simulink model "Grid_PBFORCAPF_ab_Detail_2013b_616"  (R2021b)
settings: Solver=FixedStepDiscrete  StartTime=0.0  StopTime=1.5  FixedStep=Ts_Power  RelTol=1e-3
InitFcn:
  | %% Sys Para
  | N=200;fg=50;Vbase=200;
  | Ts_Control=1/N/fg;
  | Tscon=Ts_Control;
  | Ts_Power=Ts_Control/128;
  | fsw=1/Ts_Control;
  | Vdcref=350;
  | Vdcini=Vdcref;
  | 
  | 
  | 
  | %% Load Side
  | Ll=2.0e-3;Rl=1e-2;
  | RL=100;
  | 
  | %% DG Circuit Parameters
  | %% LCL
  | L1_DG1=1.4e-3;R1=1e-3;
  | L2_DG1=0.4e-3;R2=1e-3;
  | Cx_DG1=6.3e-6;
  | 
  | L1_DG2=L1_DG1;L2_DG2=L2_DG1;Cx_DG2=Cx_DG1;
  | L1_DG3=L1_DG1;L2_DG3=L2_DG1;Cx_DG3=Cx_DG1;
  | Cdc=0.55e-3;
  | %PLL;
  | Kp_pll=88;
  | Ki_pll=0.4/Ts_Control;
  | 
  | %% DG2 Controller Parameters
  | Kpc_DG1=4.89;
  | Kic_DG1=0;
  | 
  | Kpdc_DG1=0.2;
  | Kidc_DG1=0.1;
undefined symbols (not defined in the file or in its folder): DiscIntNeverNeededParam, L2, Rd
libraries: spsThreePhaseSeriesRLCBranchLib x13, slpidlib x8, spsThreePhaseVIMeasurementLib x8, spsStairGeneratorLib x8, simulink x6, simulink_extras x6, spsSeriesRLCBranchLib x5, spsThreePhaseBreakerLib x5, spsUniversalBridgeLib x4, spsNeutralLib x4, spsGroundLib x3, spsPWMGenerator2LevelLib x3
(part 2 of 3)

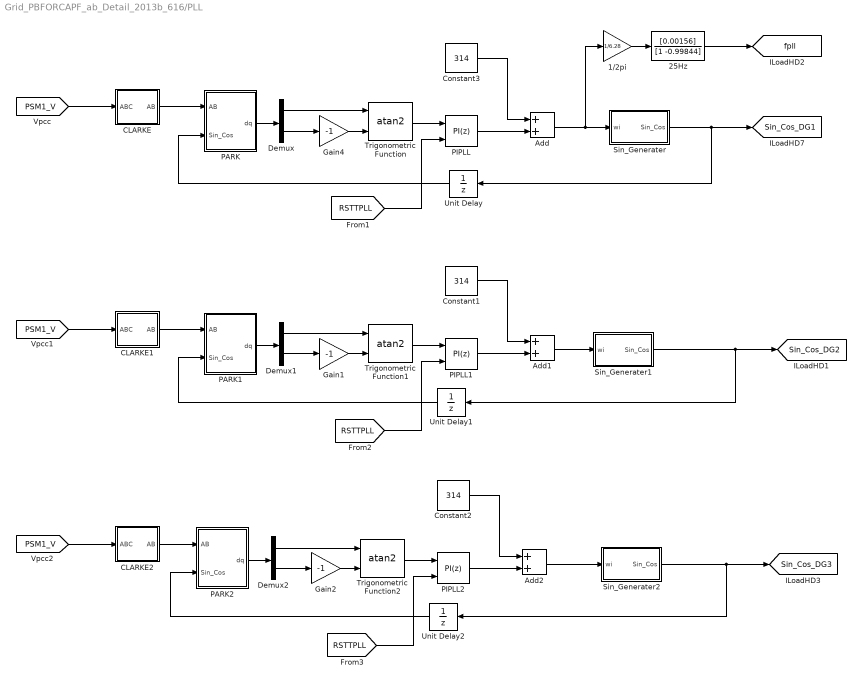
== system Grid_PBFORCAPF_ab_Detail_2013b_616/PLL ==
  1/2pi : Gain  Gain=1/6.28
  25Hz : DiscreteFilter  Numerator=[0.00156]  Denominator=[1 -0.99844]  InitialStates=50  InputProcessing=Columns as channels (frame based)  FilterStructure=Direct form II transposed
  Add : Sum
  Add1 : Sum
  Add2 : Sum
  CLARKE : Subsystem
  CLARKE1 : Subsystem
  CLARKE2 : Subsystem
  Constant1 : Constant  Value=314  SampleTime=Tscon
  Constant2 : Constant  Value=314  SampleTime=Tscon
  Constant3 : Constant  Value=314  SampleTime=Tscon
  Demux : Demux  Outputs=2
  Demux1 : Demux  Outputs=2
  Demux2 : Demux  Outputs=2
  Gain1 : Gain  Gain=-1
  Gain2 : Gain  Gain=-1
  Gain4 : Gain  Gain=-1
  PARK : Subsystem
  PARK1 : Subsystem
  PARK2 : Subsystem
  PIPLL : slpidlib/PID Controller  Controller=PI  Form=Parallel  TimeDomain=Discrete-time  UseExternalTs=off  SampleTime=-1  IntegratorMethod=Backward Euler  FilterMethod=Forward Euler  ControllerParametersSource=internal  P=Kp_pll  I=Ki_pll  D=0  N=100  UseFilter=on  TunerSelectOption=Transfer Function Based (PID Tuner App)  InitialConditionSource=internal  InitialConditionForIntegrator=0  InitialConditionForFilter=0  DifferentiatorICPrevScaledInput=0  ExternalReset=level  TrackingMode=off  Kt=1  LimitOutput=on  SatLimitsSource=internal  UpperSaturationLimit=100  LowerSaturationLimit=-100  LinearizeAsGain=off  AntiWindupMode=none  Kb=0.5  POutMin=[]  POutMax=[]  IOutMin=[]  IOutMax=[]  DOutMin=[]  DOutMax=[]  NOutMin=[]  NOutMax=[]  SumOutMin=[]  SumOutMax=[]  SaturationOutMin=[]  SaturationOutMax=[]  PParamMin=[]  PParamMax=[]  IParamMin=[]  IParamMax=[]  DParamMin=[]  DParamMax=[]  NParamMin=[]  NParamMax=[]  KbParamMin=[]  KbParamMax=[]  KtParamMin=[]  KtParamMax=[]  KbOutMin=[]  KbOutMax=[]  KtOutMin=[]  KtOutMax=[]  IntegratorOutMin=[]  IntegratorOutMax=[]  FilterOutMin=[]  FilterOutMax=[]  SumI1OutMin=[]  SumI1OutMax=[]  SumI2OutMin=[]  SumI2OutMax=[]  SumI3OutMin=[]  SumI3OutMax=[]  SumI4OutMin=[]  SumI4OutMax=[]  SumDOutMin=[]  SumDOutMax=[]  DifferentiatorOutMin=[]  DifferentiatorOutMax=[]  FilterDiffOutCoefMin=[]  FilterDiffOutCoefMax=[]  ReciprocalOutMin=[]  ReciprocalOutMax=[]  SumDenOutMin=[]  SumDenOutMax=[]  SumNumOutMin=[]  SumNumOutMax=[]  DivideOutMin=[]  DivideOutMax=[]  UdiffTsProdOutMin=[]  UdiffTsProdOutMax=[]  NTsProdOutMin=[]  NTsProdOutMax=[]  UintegralTsProdOutMin=[]  UintegralTsProdOutMax=[]  UngainTsProdOutMin=[]  UngainTsProdOutMax=[]  IntegratorContinuousStateAttributes=''  IntegratorStateMustResolveToSignalObject=off  IntegratorRTWStateStorageClass=Auto  FilterContinuousStateAttributes=''  FilterStateMustResolveToSignalObject=off  FilterRTWStateStorageClass=Auto  ParallelPVariant=InternalParameters  IdealPVariant=Disabled  IVariant=InternalParameters  DVariant=Disabled  IntegratorVariant=Discrete  SatVariant=Enabled  AWVariant=Passthrough  PCopyVariant=Disabled  TRVariant=Disabled  FdbkBlocksVariant=Forward  IdealPFdbkVariant=Disabled  SatFdbkVariant=Disabled  DerivativeFilterVariant=Disabled  NVariant=Disabled  NCopyVariant=Disabled_SignalSpec  FilterICVariant=Disabled  IntegratorICVariant=InternalICs  ExternalResetVariant=ExternalReset  TRSumVariant=Passthrough  SumFdbkVariant=Disabled  SumVariant=Sum_PI  TsampFilterVariant=InternalTs  TsampNgainVariant=Passthrough  TsampIntegralVariant=Passthrough  ExternalSaturationOutDataTypeStr=Inherit: Same as second input
      link override Integrator: IntegratorMethod=Integration: Backward Euler  gainval=1.0  ExternalReset=level  InitialConditionSource=internal  InitialCondition=InitialConditionForIntegrator  InitialConditionMode=State only (most efficient)  SampleTime=-1  OutMin=IntegratorOutMin  OutMax=IntegratorOutMax  OutDataTypeStr=IntegratorOutDataTypeStr  LimitOutput=off  UpperSaturationLimit=inf  LowerSaturationLimit=-inf  ShowSaturationPort=off  ShowStatePort=off
      link override Integrator: StateMustResolveToSignalObject=off  RTWStateStorageClass=Auto
  PIPLL1 : slpidlib/PID Controller  Controller=PI  Form=Parallel  TimeDomain=Discrete-time  UseExternalTs=off  SampleTime=-1  IntegratorMethod=Backward Euler  FilterMethod=Forward Euler  ControllerParametersSource=internal  P=Kp_pll  I=Ki_pll  D=0  N=100  UseFilter=on  TunerSelectOption=Transfer Function Based (PID Tuner App)  InitialConditionSource=internal  InitialConditionForIntegrator=0  InitialConditionForFilter=0  DifferentiatorICPrevScaledInput=0  ExternalReset=level  TrackingMode=off  Kt=1  LimitOutput=on  SatLimitsSource=internal  UpperSaturationLimit=100  LowerSaturationLimit=-100  LinearizeAsGain=off  AntiWindupMode=none  Kb=0.5  POutMin=[]  POutMax=[]  IOutMin=[]  IOutMax=[]  DOutMin=[]  DOutMax=[]  NOutMin=[]  NOutMax=[]  SumOutMin=[]  SumOutMax=[]  SaturationOutMin=[]  SaturationOutMax=[]  PParamMin=[]  PParamMax=[]  IParamMin=[]  IParamMax=[]  DParamMin=[]  DParamMax=[]  NParamMin=[]  NParamMax=[]  KbParamMin=[]  KbParamMax=[]  KtParamMin=[]  KtParamMax=[]  KbOutMin=[]  KbOutMax=[]  KtOutMin=[]  KtOutMax=[]  IntegratorOutMin=[]  IntegratorOutMax=[]  FilterOutMin=[]  FilterOutMax=[]  SumI1OutMin=[]  SumI1OutMax=[]  SumI2OutMin=[]  SumI2OutMax=[]  SumI3OutMin=[]  SumI3OutMax=[]  SumI4OutMin=[]  SumI4OutMax=[]  SumDOutMin=[]  SumDOutMax=[]  DifferentiatorOutMin=[]  DifferentiatorOutMax=[]  FilterDiffOutCoefMin=[]  FilterDiffOutCoefMax=[]  ReciprocalOutMin=[]  ReciprocalOutMax=[]  SumDenOutMin=[]  SumDenOutMax=[]  SumNumOutMin=[]  SumNumOutMax=[]  DivideOutMin=[]  DivideOutMax=[]  UdiffTsProdOutMin=[]  UdiffTsProdOutMax=[]  NTsProdOutMin=[]  NTsProdOutMax=[]  UintegralTsProdOutMin=[]  UintegralTsProdOutMax=[]  UngainTsProdOutMin=[]  UngainTsProdOutMax=[]  IntegratorContinuousStateAttributes=''  IntegratorStateMustResolveToSignalObject=off  IntegratorRTWStateStorageClass=Auto  FilterContinuousStateAttributes=''  FilterStateMustResolveToSignalObject=off  FilterRTWStateStorageClass=Auto  ParallelPVariant=InternalParameters  IdealPVariant=Disabled  IVariant=InternalParameters  DVariant=Disabled  IntegratorVariant=Discrete  SatVariant=Enabled  AWVariant=Passthrough  PCopyVariant=Disabled  TRVariant=Disabled  FdbkBlocksVariant=Forward  IdealPFdbkVariant=Disabled  SatFdbkVariant=Disabled  DerivativeFilterVariant=Disabled  NVariant=Disabled  NCopyVariant=Disabled_SignalSpec  FilterICVariant=Disabled  IntegratorICVariant=InternalICs  ExternalResetVariant=ExternalReset  TRSumVariant=Passthrough  SumFdbkVariant=Disabled  SumVariant=Sum_PI  TsampFilterVariant=InternalTs  TsampNgainVariant=Passthrough  TsampIntegralVariant=Passthrough  ExternalSaturationOutDataTypeStr=Inherit: Same as second input
      link override Integrator: IntegratorMethod=Integration: Backward Euler  gainval=1.0  ExternalReset=level  InitialConditionSource=internal  InitialCondition=InitialConditionForIntegrator  InitialConditionMode=State only (most efficient)  SampleTime=-1  OutMin=IntegratorOutMin  OutMax=IntegratorOutMax  OutDataTypeStr=IntegratorOutDataTypeStr  LimitOutput=off  UpperSaturationLimit=inf  LowerSaturationLimit=-inf  ShowSaturationPort=off  ShowStatePort=off
      link override Integrator: StateMustResolveToSignalObject=off  RTWStateStorageClass=Auto
  PIPLL2 : slpidlib/PID Controller  Controller=PI  Form=Parallel  TimeDomain=Discrete-time  UseExternalTs=off  SampleTime=-1  IntegratorMethod=Backward Euler  FilterMethod=Forward Euler  ControllerParametersSource=internal  P=Kp_pll  I=Ki_pll  D=0  N=100  UseFilter=on  TunerSelectOption=Transfer Function Based (PID Tuner App)  InitialConditionSource=internal  InitialConditionForIntegrator=0  InitialConditionForFilter=0  DifferentiatorICPrevScaledInput=0  ExternalReset=level  TrackingMode=off  Kt=1  LimitOutput=on  SatLimitsSource=internal  UpperSaturationLimit=100  LowerSaturationLimit=-100  LinearizeAsGain=off  AntiWindupMode=none  Kb=0.5  POutMin=[]  POutMax=[]  IOutMin=[]  IOutMax=[]  DOutMin=[]  DOutMax=[]  NOutMin=[]  NOutMax=[]  SumOutMin=[]  SumOutMax=[]  SaturationOutMin=[]  SaturationOutMax=[]  PParamMin=[]  PParamMax=[]  IParamMin=[]  IParamMax=[]  DParamMin=[]  DParamMax=[]  NParamMin=[]  NParamMax=[]  KbParamMin=[]  KbParamMax=[]  KtParamMin=[]  KtParamMax=[]  KbOutMin=[]  KbOutMax=[]  KtOutMin=[]  KtOutMax=[]  IntegratorOutMin=[]  IntegratorOutMax=[]  FilterOutMin=[]  FilterOutMax=[]  SumI1OutMin=[]  SumI1OutMax=[]  SumI2OutMin=[]  SumI2OutMax=[]  SumI3OutMin=[]  SumI3OutMax=[]  SumI4OutMin=[]  SumI4OutMax=[]  SumDOutMin=[]  SumDOutMax=[]  DifferentiatorOutMin=[]  DifferentiatorOutMax=[]  FilterDiffOutCoefMin=[]  FilterDiffOutCoefMax=[]  ReciprocalOutMin=[]  ReciprocalOutMax=[]  SumDenOutMin=[]  SumDenOutMax=[]  SumNumOutMin=[]  SumNumOutMax=[]  DivideOutMin=[]  DivideOutMax=[]  UdiffTsProdOutMin=[]  UdiffTsProdOutMax=[]  NTsProdOutMin=[]  NTsProdOutMax=[]  UintegralTsProdOutMin=[]  UintegralTsProdOutMax=[]  UngainTsProdOutMin=[]  UngainTsProdOutMax=[]  IntegratorContinuousStateAttributes=''  IntegratorStateMustResolveToSignalObject=off  IntegratorRTWStateStorageClass=Auto  FilterContinuousStateAttributes=''  FilterStateMustResolveToSignalObject=off  FilterRTWStateStorageClass=Auto  ParallelPVariant=InternalParameters  IdealPVariant=Disabled  IVariant=InternalParameters  DVariant=Disabled  IntegratorVariant=Discrete  SatVariant=Enabled  AWVariant=Passthrough  PCopyVariant=Disabled  TRVariant=Disabled  FdbkBlocksVariant=Forward  IdealPFdbkVariant=Disabled  SatFdbkVariant=Disabled  DerivativeFilterVariant=Disabled  NVariant=Disabled  NCopyVariant=Disabled_SignalSpec  FilterICVariant=Disabled  IntegratorICVariant=InternalICs  ExternalResetVariant=ExternalReset  TRSumVariant=Passthrough  SumFdbkVariant=Disabled  SumVariant=Sum_PI  TsampFilterVariant=InternalTs  TsampNgainVariant=Passthrough  TsampIntegralVariant=Passthrough  ExternalSaturationOutDataTypeStr=Inherit: Same as second input
      link override Integrator: IntegratorMethod=Integration: Backward Euler  gainval=1.0  ExternalReset=level  InitialConditionSource=internal  InitialCondition=InitialConditionForIntegrator  InitialConditionMode=State only (most efficient)  SampleTime=-1  OutMin=IntegratorOutMin  OutMax=IntegratorOutMax  OutDataTypeStr=IntegratorOutDataTypeStr  LimitOutput=off  UpperSaturationLimit=inf  LowerSaturationLimit=-inf  ShowSaturationPort=off  ShowStatePort=off
      link override Integrator: StateMustResolveToSignalObject=off  RTWStateStorageClass=Auto
  Sin_Generater : Subsystem
  Sin_Generater1 : Subsystem
  Sin_Generater2 : Subsystem
  Trigonometric Function : Trigonometry  Operator=atan2
  Trigonometric Function1 : Trigonometry  Operator=atan2
  Trigonometric Function2 : Trigonometry  Operator=atan2
  Unit Delay : UnitDelay  SampleTime=-1  HasFrameUpgradeWarning=on
  Unit Delay1 : UnitDelay  SampleTime=-1  HasFrameUpgradeWarning=on
  Unit Delay2 : UnitDelay  SampleTime=-1  HasFrameUpgradeWarning=on
  tag scope: Sin_Cos_DG1=global, Sin_Cos_DG2=global, Sin_Cos_DG3=global, fpll=global
  wires:
  Gain4/1 -> Trigonometric Function/2
  Demux/2 -> Gain4/1
  Demux/1 -> Trigonometric Function/1
  Trigonometric Function/1 -> PIPLL/1
  PIPLL/1 -> Add/2
  Constant3/1 -> Add/1
  CLARKE/1(AB) -> PARK/1(AB)
  Add/1 -> 1/2pi/1, Sin_Generater/1(wi)
  Sin_Generater/1(Sin_Cos) -> [Sin_Cos_DG1], Unit Delay/1
  PARK/1(dq) -> Demux/1
  Unit Delay/1 -> PARK/2(Sin_Cos)
  [PSM1_V] -> CLARKE/1(ABC)
  [RSTTPLL] -> PIPLL/2
  [RSTTPLL] -> PIPLL1/2
  [PSM1_V] -> CLARKE1/1(ABC)
  Unit Delay1/1 -> PARK1/2(Sin_Cos)
  PARK1/1(dq) -> Demux1/1
  Sin_Generater1/1(Sin_Cos) -> Unit Delay1/1, [Sin_Cos_DG2]
  Add1/1 -> Sin_Generater1/1(wi)
  CLARKE1/1(AB) -> PARK1/1(AB)
  Constant1/1 -> Add1/1
  PIPLL1/1 -> Add1/2
  Trigonometric Function1/1 -> PIPLL1/1
  Demux1/1 -> Trigonometric Function1/1
  Demux1/2 -> Gain1/1
  Gain1/1 -> Trigonometric Function1/2
  Gain2/1 -> Trigonometric Function2/2
  Demux2/2 -> Gain2/1
  Demux2/1 -> Trigonometric Function2/1
  Trigonometric Function2/1 -> PIPLL2/1
  PIPLL2/1 -> Add2/2
  Constant2/1 -> Add2/1
  CLARKE2/1(AB) -> PARK2/1(AB)
  Add2/1 -> Sin_Generater2/1(wi)
  Sin_Generater2/1(Sin_Cos) -> [Sin_Cos_DG3], Unit Delay2/1
  PARK2/1(dq) -> Demux2/1
  Unit Delay2/1 -> PARK2/2(Sin_Cos)
  [PSM1_V] -> CLARKE2/1(ABC)
  [RSTTPLL] -> PIPLL2/2
  25Hz/1 -> [fpll]
  1/2pi/1 -> 25Hz/1

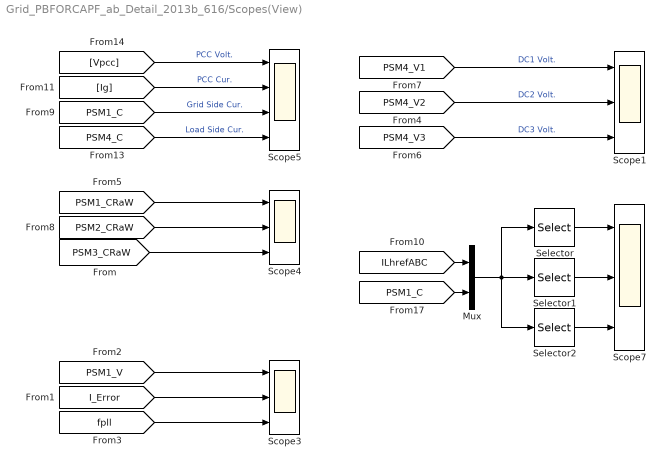
== system Grid_PBFORCAPF_ab_Detail_2013b_616/Scopes(View) ==
  Mux : Mux  Inputs=2
  Scope{1,3..4,7} (4 alike) : Scope  NumInputPorts=3
  Scope5 : Scope  NumInputPorts=4
  Selector : Selector  InputPortWidth=6  IndexOptions=Index vector (dialog)  Indices=[1 4]  OutputSizes=1
  Selector1 : Selector  InputPortWidth=6  IndexOptions=Index vector (dialog)  Indices=[2 5]  OutputSizes=1
  Selector2 : Selector  InputPortWidth=6  IndexOptions=Index vector (dialog)  Indices=[3 6]  OutputSizes=1
  wires:
  [I_Error] -> Scope3/2
  [PSM1_V] -> Scope3/1
  [PSM1_CRaW] -> Scope4/1
  [PSM2_CRaW] -> Scope4/2
  [Ig] -> Scope5/2  "PCC Cur."
  [PSM1_C] -> Mux/2
  Mux/1 -> Selector/1, Selector2/1, Selector1/1
  Selector/1 -> Scope7/1
  Selector2/1 -> Scope7/3
  [ILhrefABC] -> Mux/1
  Selector1/1 -> Scope7/2
  [PSM1_C] -> Scope5/3  "Grid Side Cur."
  [Vpcc] -> Scope5/1  "PCC Volt."
  [PSM4_C] -> Scope5/4  "Load Side Cur."
  [PSM3_CRaW] -> Scope4/3
  [fpll] -> Scope3/3
  [PSM4_V1] -> Scope1/1  "DC1 Volt."
  [PSM4_V2] -> Scope1/2  "DC2 Volt."
  [PSM4_V3] -> Scope1/3  "DC3 Volt."

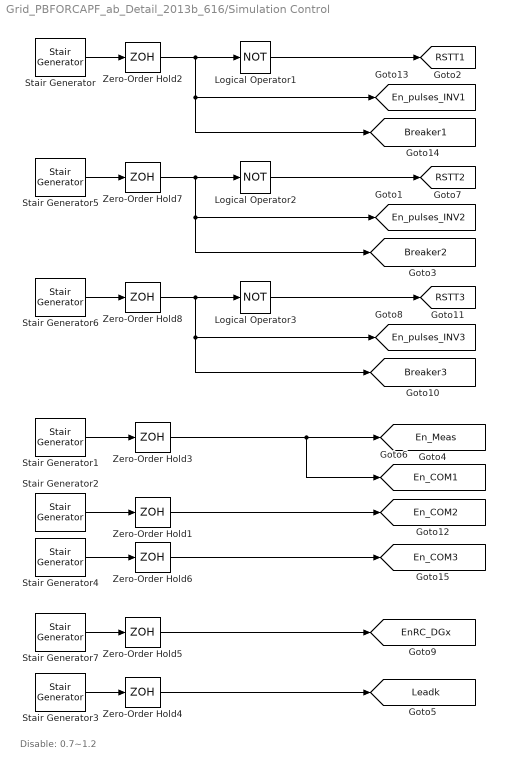
== system Grid_PBFORCAPF_ab_Detail_2013b_616/Simulation Control ==
  note: Disable: 0.7~1.2
  Logical Operator1 : Logic  Operator=NOT  IconShape=distinctive  AllPortsSameDT=off  OutDataTypeStr=boolean
  Logical Operator2 : Logic  Operator=NOT  IconShape=distinctive  AllPortsSameDT=off  OutDataTypeStr=boolean
  Logical Operator3 : Logic  Operator=NOT  IconShape=distinctive  AllPortsSameDT=off  OutDataTypeStr=boolean
  Stair Generator : spsStairGeneratorLib/Stair Generator  t=[0, 0.1]  e=[0, 1]  Ts=0
  Stair Generator1 : spsStairGeneratorLib/Stair Generator  t=[0 0.2]  e=[0 1.0]  Ts=0
  Stair Generator2 : spsStairGeneratorLib/Stair Generator  t=[0 0.8]  e=[0 0.333]  Ts=0
  Stair Generator3 : spsStairGeneratorLib/Stair Generator  t=[0 0.3 0.5]  e=[3 3 3]%[2 3 4 ]%  Ts=0
  Stair Generator4 : spsStairGeneratorLib/Stair Generator  t=[0 1]  e=[0 0.333]  Ts=0
  Stair Generator5 : spsStairGeneratorLib/Stair Generator  t=[0, 0.3]  e=[0, 1]  Ts=0
  Stair Generator6 : spsStairGeneratorLib/Stair Generator  t=[0, 0.5]  e=[0, 1]  Ts=0
  Stair Generator7 : spsStairGeneratorLib/Stair Generator  t=[0 0.2]  e=[0 1]  Ts=0
  Zero-Order Hold{1..8} (8 alike) : ZeroOrderHold  SampleTime=Ts_Control
  tag scope: Breaker1=global, Breaker2=global, Breaker3=global, EnRC_DGx=global, En_COM1=global, En_COM2=global, En_COM3=global, En_Meas=global, En_pulses_INV1=global, En_pulses_INV2=global, En_pulses_INV3=global, Leadk=global, RSTT1=global, RSTT2=global, RSTT3=global
  wires:
  Stair Generator/1 -> Zero-Order Hold2/1
  Zero-Order Hold2/1 -> [Breaker1], [En_pulses_INV1], Logical Operator1/1
  Logical Operator1/1 -> [RSTT1]
  Stair Generator7/1 -> Zero-Order Hold5/1
  Zero-Order Hold5/1 -> [EnRC_DGx]
  Stair Generator3/1 -> Zero-Order Hold4/1
  Zero-Order Hold4/1 -> [Leadk]
  Zero-Order Hold3/1 -> [En_COM1], [En_Meas]
  Stair Generator1/1 -> Zero-Order Hold3/1
  Stair Generator2/1 -> Zero-Order Hold1/1
  Zero-Order Hold1/1 -> [En_COM2]
  Zero-Order Hold6/1 -> [En_COM3]
  Stair Generator4/1 -> Zero-Order Hold6/1
  Logical Operator2/1 -> [RSTT2]
  Zero-Order Hold7/1 -> Logical Operator2/1, [En_pulses_INV2], [Breaker2]
  Stair Generator5/1 -> Zero-Order Hold7/1
  Stair Generator6/1 -> Zero-Order Hold8/1
  Zero-Order Hold8/1 -> [Breaker3], [En_pulses_INV3], Logical Operator3/1
  Logical Operator3/1 -> [RSTT3]

== system Grid_PBFORCAPF_ab_Detail_2013b_616/Controller1/CLARKE1 ==
  ABC : Inport
  Fcn : Fcn  Expr=2/3*(u(1)-u(2)/2-u(3)/2)
  Fcn1 : Fcn  Expr=(u(2)-u(3))/sqrt(3)
  Mux : Mux  Inputs=2
  AB : Outport  VectorParamsAs1DForOutWhenUnconnected=off
  wires:
  Mux/1 -> AB/1
  Fcn1/1 -> Mux/2  "beta"
  Fcn/1 -> Mux/1  "alfa"
  ABC/1 -> Fcn/1, Fcn1/1

== system Grid_PBFORCAPF_ab_Detail_2013b_616/Controller1/CLARKE2 ==
  ABC : Inport
  Fcn : Fcn  Expr=2/3*(u(1)-u(2)/2-u(3)/2)
  Fcn1 : Fcn  Expr=(u(2)-u(3))/sqrt(3)
  Mux : Mux  Inputs=2
  AB : Outport  VectorParamsAs1DForOutWhenUnconnected=off
  wires:
  ABC/1 -> Fcn1/1, Fcn/1
  Fcn/1 -> Mux/1  "alfa"
  Fcn1/1 -> Mux/2  "beta"
  Mux/1 -> AB/1

== system Grid_PBFORCAPF_ab_Detail_2013b_616/Controller1/DSOGI ==
  In : Inport
  QSOGI : Subsystem  mask{h=h, KIh=KIh, wc=wc, phch=phch, Ts=Ts}
      mask prompts: h "Selected harmonic orders"; KIh "Integral gain of QSOGI"; wc "Inversion of maximum gain"; phch "Phase compensation angle"; Ts "Sampling Period"
      mask Display: disp('QSOGIh(z)')
  Out : Outport  VectorParamsAs1DForOutWhenUnconnected=off
  wires:
  QSOGI/1(vh) -> Out/1
  In/1 -> QSOGI/1(v)

== system Grid_PBFORCAPF_ab_Detail_2013b_616/Controller1/FORCAB ==
  In : Inport
  f1 : Inport  Port=2
  Rest : Inport  Port=3
  Bias1 : Constant  Value=0
  Delay : Delay  DelayLength=100
  Discrete FIR : DiscreteFir  Coefficients=[0.25 0.5 0.25]
  Discrete Filter1 : DiscreteFilter  Numerator=[0.001]  Denominator=[1 -0.999]
  Gain1 : Gain  Gain=Q
  Mux : Mux  Inputs=2
  Ni--Lead : Fcn  Expr=u(1)-u(2)-101
  Saturation2 : Saturate  UpperLimit=300  LowerLimit=50
  Saturation3 : Saturate  UpperLimit=1  LowerLimit=0
  Seperated1 : Subsystem
  Subsystem1 : Subsystem
      mask Display: disp('z^(-F)');
  Sum18 : Sum  Inputs=|++
  Sum4 : Sum  Inputs=-+
  Switch : Switch  Threshold=0.001
  Variable Integer Delay : Delay  DelayLengthSource=Input port  DelayLengthUpperLimit=300
      settings: InputPortMap=u0,p1
  Variable Integer Delay1 : Delay  DelayLengthSource=Input port  DelayLengthUpperLimit=300
      settings: InputPortMap=u0,p1
  Out : Outport  VectorParamsAs1DForOutWhenUnconnected=off
  wires:
  Sum18/1 -> Variable Integer Delay/1
  In/1 -> Sum18/1
  Switch/1 -> Discrete FIR/1
  Bias1/1 -> Switch/3
  Rest/1 -> Switch/2
  [Leadk] -> Mux/2, Variable Integer Delay1/2
  Variable Integer Delay/1 -> Delay/1
  Ni--Lead/1 -> Variable Integer Delay/2
  Gain1/1 -> Subsystem1/1(In), Out/1
  Variable Integer Delay1/1 -> Sum18/2
  Discrete FIR/1 -> Gain1/1
  Saturation3/1 -> Discrete Filter1/1
  Seperated1/2(N) -> Sum4/2
  Saturation2/1 -> Mux/1, Sum4/1  "Ni"
  Sum4/1 -> Saturation3/1  "F"
  Seperated1/1(Ni) -> Saturation2/1
  f1/1 -> Seperated1/1(fi)
  Subsystem1/1(Out) -> Variable Integer Delay1/1
  Discrete Filter1/1 -> Subsystem1/2(F)
  Mux/1 -> Ni--Lead/1
  Delay/1 -> Switch/1

== system Grid_PBFORCAPF_ab_Detail_2013b_616/Controller1/ICLARKE1 ==
  AB : Inport
  -0.5alfa+sqrt(3)/2*beta : Fcn  Expr=-u(1)/2+u(2)*sqrt(3)/2
  "-0.5alfa-sqrt(3)/2*beta " : Fcn  Expr=-u(1)/2-u(2)*sqrt(3)/2
  Mux3 : Mux  Inputs=3
  a=alfa : Fcn  Expr=u(1)
  ABC : Outport  VectorParamsAs1DForOutWhenUnconnected=off
  wires:
  -0.5alfa+sqrt(3)/2*beta/1 -> Mux3/2  "b"
  "-0.5alfa-sqrt(3)/2*beta "/1 -> Mux3/3  "c"
  Mux3/1 -> ABC/1
  AB/1 -> "-0.5alfa-sqrt(3)/2*beta "/1, -0.5alfa+sqrt(3)/2*beta/1, a=alfa/1
  a=alfa/1 -> Mux3/1  "a"

== system Grid_PBFORCAPF_ab_Detail_2013b_616/Controller1/SV Modulator Pattern #1 ==
  note: m_max
  note: 6/pi(2/sqrt(3)-1)=0.295
  Valphabeta : Inport
  Cartesian to Polar : simulink_extras/Transformations/Cartesian to Polar
  "Compute time duration of switching states (Ta,Tb,To) " : Subsystem
  Constant : Constant  Value=pi/3
  Constant2 : Constant  Value=2*pi
  Demux : Demux  Outputs=2
  "Determine the sector of U* based on alpha (rad). Also, determine if the sector number is odd" : Subsystem
  Generate pulse pattern : Subsystem
      mask init:
      | %Switching pattern:
      | pat1=[0 1 1 1 1 1 0;0 0 1 1 1 0 0;0 0 0 1 0 0 0];
      | pat1(:,:,2)=[0 0 1 1 1 0 0;0 1 1 1 1 1 0;0 0 0 1 0 0 0];
      | pat1(:,:,3)=[0 0 0 1 0 0 0;0 1 1 1 1 1 0;0 0 1 1 1 0 0];
      | pat1(:,:,4)=[0 0 0 1 0 0 0;0 0 1 1 1 0 0;0 1 1 1 1 1 0];
      | pat1(:,:,5)=[0 0 1 1 1 0 0;0 0 0 1 0 0 0;0 1 1 1 1 1 0];
      | pat1(:,:,6)=[0 1 1 1 1 1 0;0 0 0 1 0 0 0;0 0 1 1 1 0 0];
  Hexagonal : Saturate  UpperLimit=0  LowerLimit=-10
  INFO : Subsystem
      mask Display: disp('?')
  Math Function : Math  Operator=reciprocal  SignedPower=on  SaturateOnIntegerOverflow=on
  Math Function2 : Math  Operator=mod  SignedPower=on  SaturateOnIntegerOverflow=on
  Mux : Mux  Inputs=2
  Polar to Cartesian : simulink_extras/Transformations/Polar to Cartesian
      settings: SourceProductBaseCode=SL
  Saturation : Saturate  UpperLimit=6  LowerLimit=1
  Subsystem : Subsystem
  Sum1 : Sum  Inputs=+-  SaturateOnIntegerOverflow=on
  Sum2 : Sum  SaturateOnIntegerOverflow=on
  Sum3 : Sum  SaturateOnIntegerOverflow=on
  Trigonometric Function : Trigonometry
  Dabc : Outport  VectorParamsAs1DForOutWhenUnconnected=off
  tag scope: Vsatab_DG1=global, Vunsatab_DG1=global
  wires:
  Math Function2/1 -> Polar to Cartesian/2, "Compute time duration of switching states (Ta,Tb,To) "/1(alpha), "Determine the sector of U* based on alpha (rad). Also, determine if the sector number is odd"/1(alpha)
  Generate pulse pattern/1(abc) -> Dabc/1
  "Compute time duration of switching states (Ta,Tb,To) "/1(Ta_Tb_To) -> Subsystem/1(TaTbTo)
  "Determine the sector of U* based on alpha (rad). Also, determine if the sector number is odd"/2(Odd_S) -> "Compute time duration of switching states (Ta,Tb,To) "/4(Odd_S)
  "Determine the sector of U* based on alpha (rad). Also, determine if the sector number is odd"/1(Sn) -> Saturation/1, "Compute time duration of switching states (Ta,Tb,To) "/3(Sn)
  Subsystem/1(D1D2D0) -> Generate pulse pattern/2(D120)
  Saturation/1 -> Generate pulse pattern/1(Sn)
  Demux/1 -> Cartesian to Polar/1
  Demux/2 -> Cartesian to Polar/2
  Cartesian to Polar/2 -> Math Function2/1
  Cartesian to Polar/1 -> Sum2/2, Sum1/2
  Constant2/1 -> Math Function2/2
  Sum2/1 -> Polar to Cartesian/1, "Compute time duration of switching states (Ta,Tb,To) "/2(m)
  Constant/1 -> Sum3/2
  [alpha] -> Sum3/1
  Trigonometric Function/1 -> Math Function/1
  Sum1/1 -> Hexagonal/1
  Hexagonal/1 -> Sum2/1
  Polar to Cartesian/2 -> Mux/2
  Polar to Cartesian/1 -> Mux/1
  Mux/1 -> [Vsatab_DG1]
  Sum3/1 -> Trigonometric Function/1
  Math Function/1 -> Sum1/1
  Valphabeta/1 -> [Vunsatab_DG1], Demux/1

== system Grid_PBFORCAPF_ab_Detail_2013b_616/Controller2/CLARKE1 ==
  ABC : Inport
  Fcn : Fcn  Expr=2/3*(u(1)-u(2)/2-u(3)/2)
  Fcn1 : Fcn  Expr=(u(2)-u(3))/sqrt(3)
  Mux : Mux  Inputs=2
  AB : Outport  VectorParamsAs1DForOutWhenUnconnected=off
  wires:
  ABC/1 -> Fcn1/1, Fcn/1
  Fcn/1 -> Mux/1  "alfa"
  Fcn1/1 -> Mux/2  "beta"
  Mux/1 -> AB/1

== system Grid_PBFORCAPF_ab_Detail_2013b_616/Controller2/CLARKE2 ==
  ABC : Inport
  Fcn : Fcn  Expr=2/3*(u(1)-u(2)/2-u(3)/2)
  Fcn1 : Fcn  Expr=(u(2)-u(3))/sqrt(3)
  Mux : Mux  Inputs=2
  AB : Outport  VectorParamsAs1DForOutWhenUnconnected=off
  wires:
  Mux/1 -> AB/1
  Fcn1/1 -> Mux/2  "beta"
  Fcn/1 -> Mux/1  "alfa"
  ABC/1 -> Fcn/1, Fcn1/1

== system Grid_PBFORCAPF_ab_Detail_2013b_616/Controller2/DSOGI ==
  In : Inport
  QSOGI : Subsystem  mask{h=h, KIh=KIh, wc=wc, phch=phch, Ts=Ts}
      mask prompts: h "Selected harmonic orders"; KIh "Integral gain of QSOGI"; wc "Inversion of maximum gain"; phch "Phase compensation angle"; Ts "Sampling Period"
      mask Display: disp('QSOGIh(z)')
  Out : Outport  VectorParamsAs1DForOutWhenUnconnected=off
  wires:
  In/1 -> QSOGI/1(v)
  QSOGI/1(vh) -> Out/1

== system Grid_PBFORCAPF_ab_Detail_2013b_616/Controller2/FORCAB ==
  In : Inport
  f1 : Inport  Port=2
  Rest : Inport  Port=3
  Bias1 : Constant  Value=0
  Discrete FIR : DiscreteFir  Coefficients=[0.25 0.5 0.25]
  Discrete Filter1 : DiscreteFilter  Numerator=[0.001]  Denominator=[1 -0.999]
  Gain1 : Gain  Gain=Q
  Mux : Mux  Inputs=2
  Ni--Lead : Fcn  Expr=u(1)-u(2)-1
  Saturation2 : Saturate  UpperLimit=300  LowerLimit=50
  Saturation3 : Saturate  UpperLimit=1  LowerLimit=0
  Seperated1 : Subsystem
  Subsystem1 : Subsystem
      mask Display: disp('z^(-F)');
  Sum18 : Sum  Inputs=|++
  Sum4 : Sum  Inputs=-+
  Switch : Switch  Threshold=0.001
  Variable Integer Delay : Delay  DelayLengthSource=Input port  DelayLengthUpperLimit=300
      settings: InputPortMap=u0,p1
  Variable Integer Delay1 : Delay  DelayLengthSource=Input port  DelayLengthUpperLimit=300
      settings: InputPortMap=u0,p1
  Out : Outport  VectorParamsAs1DForOutWhenUnconnected=off
  wires:
  Mux/1 -> Ni--Lead/1
  Discrete Filter1/1 -> Subsystem1/2(F)
  Subsystem1/1(Out) -> Variable Integer Delay1/1
  f1/1 -> Seperated1/1(fi)
  Seperated1/1(Ni) -> Saturation2/1
  Sum4/1 -> Saturation3/1  "F"
  Saturation2/1 -> Sum4/1, Mux/1  "Ni"
  Seperated1/2(N) -> Sum4/2
  Saturation3/1 -> Discrete Filter1/1
  Discrete FIR/1 -> Gain1/1
  Variable Integer Delay1/1 -> Sum18/2
  Gain1/1 -> Out/1, Subsystem1/1(In)
  Ni--Lead/1 -> Variable Integer Delay/2
  Variable Integer Delay/1 -> Switch/1
  [Leadk] -> Variable Integer Delay1/2, Mux/2
  Rest/1 -> Switch/2
  Bias1/1 -> Switch/3
  Switch/1 -> Discrete FIR/1
  In/1 -> Sum18/1
  Sum18/1 -> Variable Integer Delay/1

== system Grid_PBFORCAPF_ab_Detail_2013b_616/Controller2/ICLARKE1 ==
  AB : Inport
  -0.5alfa+sqrt(3)/2*beta : Fcn  Expr=-u(1)/2+u(2)*sqrt(3)/2
  "-0.5alfa-sqrt(3)/2*beta " : Fcn  Expr=-u(1)/2-u(2)*sqrt(3)/2
  Mux3 : Mux  Inputs=3
  a=alfa : Fcn  Expr=u(1)
  ABC : Outport  VectorParamsAs1DForOutWhenUnconnected=off
  wires:
  a=alfa/1 -> Mux3/1  "a"
  AB/1 -> a=alfa/1, -0.5alfa+sqrt(3)/2*beta/1, "-0.5alfa-sqrt(3)/2*beta "/1
  Mux3/1 -> ABC/1
  "-0.5alfa-sqrt(3)/2*beta "/1 -> Mux3/3  "c"
  -0.5alfa+sqrt(3)/2*beta/1 -> Mux3/2  "b"

== system Grid_PBFORCAPF_ab_Detail_2013b_616/Controller2/IPARK ==
  dq : Inport
  Sin_Cos : Inport  Port=2
  Mux1 : Mux  Inputs=2
  Mux2 : Mux  Inputs=2
  cos*d-sin*q : Fcn  Expr=u(1)*u(4)-u(2)*u(3)
  sin*d+cos*q : Fcn  Expr=u(1)*u(3)+u(2)*u(4)
  AB : Outport  VectorParamsAs1DForOutWhenUnconnected=off
  wires:
  Mux1/1 -> AB/1
  sin*d+cos*q/1 -> Mux1/2  "beta"
  cos*d-sin*q/1 -> Mux1/1
  dq/1 -> Mux2/1
  Sin_Cos/1 -> Mux2/2
  Mux2/1 -> sin*d+cos*q/1, cos*d-sin*q/1

== system Grid_PBFORCAPF_ab_Detail_2013b_616/Controller2/SV Modulator Pattern #1 ==
  note: 6/pi(2/sqrt(3)-1)=0.295
  note: m_max
  Valphabeta : Inport
  Cartesian to Polar : simulink_extras/Transformations/Cartesian to Polar
  "Compute time duration of switching states (Ta,Tb,To) " : Subsystem
  Constant : Constant  Value=pi/3
  Constant2 : Constant  Value=2*pi
  Demux : Demux  Outputs=2
  "Determine the sector of U* based on alpha (rad). Also, determine if the sector number is odd" : Subsystem
  Generate pulse pattern : Subsystem
      mask init: same as Grid_PBFORCAPF_ab_Detail_2013b_616/Controller1/SV Modulator Pattern #1/Generate pulse pattern
  Hexagonal : Saturate  UpperLimit=0  LowerLimit=-10
  INFO : Subsystem
      mask Display: disp('?')
  Math Function : Math  Operator=reciprocal  SignedPower=on  SaturateOnIntegerOverflow=on
  Math Function2 : Math  Operator=mod  SignedPower=on  SaturateOnIntegerOverflow=on
  Mux : Mux  Inputs=2
  Polar to Cartesian : simulink_extras/Transformations/Polar to Cartesian
      settings: SourceProductBaseCode=SL
  Saturation : Saturate  UpperLimit=6  LowerLimit=1
  Subsystem : Subsystem
  Sum1 : Sum  Inputs=+-  SaturateOnIntegerOverflow=on
  Sum2 : Sum  SaturateOnIntegerOverflow=on
  Sum3 : Sum  SaturateOnIntegerOverflow=on
  Trigonometric Function : Trigonometry
  Dabc : Outport  VectorParamsAs1DForOutWhenUnconnected=off
  tag scope: Vsatab_DG2=global, Vunsatab_DG2=global
  wires:
  Valphabeta/1 -> Demux/1, [Vunsatab_DG2]
  Math Function/1 -> Sum1/1
  Sum3/1 -> Trigonometric Function/1
  Mux/1 -> [Vsatab_DG2]
  Polar to Cartesian/1 -> Mux/1
  Polar to Cartesian/2 -> Mux/2
  Hexagonal/1 -> Sum2/1
  Sum1/1 -> Hexagonal/1
  Trigonometric Function/1 -> Math Function/1
  [alpha2] -> Sum3/1
  Constant/1 -> Sum3/2
  Sum2/1 -> "Compute time duration of switching states (Ta,Tb,To) "/2(m), Polar to Cartesian/1
  Constant2/1 -> Math Function2/2
  Cartesian to Polar/1 -> Sum1/2, Sum2/2
  Cartesian to Polar/2 -> Math Function2/1
  Demux/2 -> Cartesian to Polar/2
  Demux/1 -> Cartesian to Polar/1
  Saturation/1 -> Generate pulse pattern/1(Sn)
  Subsystem/1(D1D2D0) -> Generate pulse pattern/2(D120)
  "Determine the sector of U* based on alpha (rad). Also, determine if the sector number is odd"/1(Sn) -> "Compute time duration of switching states (Ta,Tb,To) "/3(Sn), Saturation/1
  "Determine the sector of U* based on alpha (rad). Also, determine if the sector number is odd"/2(Odd_S) -> "Compute time duration of switching states (Ta,Tb,To) "/4(Odd_S)
  "Compute time duration of switching states (Ta,Tb,To) "/1(Ta_Tb_To) -> Subsystem/1(TaTbTo)
  Generate pulse pattern/1(abc) -> Dabc/1
  Math Function2/1 -> "Determine the sector of U* based on alpha (rad). Also, determine if the sector number is odd"/1(alpha), "Compute time duration of switching states (Ta,Tb,To) "/1(alpha), Polar to Cartesian/2

== system Grid_PBFORCAPF_ab_Detail_2013b_616/Controller3/CLARKE1 ==
  ABC : Inport
  Fcn : Fcn  Expr=2/3*(u(1)-u(2)/2-u(3)/2)
  Fcn1 : Fcn  Expr=(u(2)-u(3))/sqrt(3)
  Mux : Mux  Inputs=2
  AB : Outport  VectorParamsAs1DForOutWhenUnconnected=off
  wires:
  Mux/1 -> AB/1
  Fcn1/1 -> Mux/2  "beta"
  Fcn/1 -> Mux/1  "alfa"
  ABC/1 -> Fcn/1, Fcn1/1

== system Grid_PBFORCAPF_ab_Detail_2013b_616/Controller3/CLARKE2 ==
  ABC : Inport
  Fcn : Fcn  Expr=2/3*(u(1)-u(2)/2-u(3)/2)
  Fcn1 : Fcn  Expr=(u(2)-u(3))/sqrt(3)
  Mux : Mux  Inputs=2
  AB : Outport  VectorParamsAs1DForOutWhenUnconnected=off
  wires:
  ABC/1 -> Fcn1/1, Fcn/1
  Fcn/1 -> Mux/1  "alfa"
  Fcn1/1 -> Mux/2  "beta"
  Mux/1 -> AB/1

== system Grid_PBFORCAPF_ab_Detail_2013b_616/Controller3/DSOGI ==
  In : Inport
  QSOGI : Subsystem  mask{h=h, KIh=KIh, wc=wc, phch=phch, Ts=Ts}
      mask prompts: h "Selected harmonic orders"; KIh "Integral gain of QSOGI"; wc "Inversion of maximum gain"; phch "Phase compensation angle"; Ts "Sampling Period"
      mask Display: disp('QSOGIh(z)')
  Out : Outport  VectorParamsAs1DForOutWhenUnconnected=off
  wires:
  QSOGI/1(vh) -> Out/1
  In/1 -> QSOGI/1(v)

== system Grid_PBFORCAPF_ab_Detail_2013b_616/Controller3/FORCAB ==
  In : Inport
  f1 : Inport  Port=2
  Rest : Inport  Port=3
  Bias1 : Constant  Value=0
  Discrete FIR : DiscreteFir  Coefficients=[0.25 0.5 0.25]
  Discrete Filter1 : DiscreteFilter  Numerator=[0.001]  Denominator=[1 -0.999]
  Gain1 : Gain  Gain=Q
  Mux : Mux  Inputs=2
  Ni--Lead : Fcn  Expr=u(1)-u(2)-1
  Saturation2 : Saturate  UpperLimit=300  LowerLimit=50
  Saturation3 : Saturate  UpperLimit=1  LowerLimit=0
  Seperated1 : Subsystem
  Subsystem1 : Subsystem
      mask Display: disp('z^(-F)');
  Sum18 : Sum  Inputs=|++
  Sum4 : Sum  Inputs=-+
  Switch : Switch  Threshold=0.001
  Variable Integer Delay : Delay  DelayLengthSource=Input port  DelayLengthUpperLimit=300
      settings: InputPortMap=u0,p1
  Variable Integer Delay1 : Delay  DelayLengthSource=Input port  DelayLengthUpperLimit=300
      settings: InputPortMap=u0,p1
  Out : Outport  VectorParamsAs1DForOutWhenUnconnected=off
  wires:
  Sum18/1 -> Variable Integer Delay/1
  In/1 -> Sum18/1
  Switch/1 -> Discrete FIR/1
  Bias1/1 -> Switch/3
  Rest/1 -> Switch/2
  [Leadk] -> Mux/2, Variable Integer Delay1/2
  Variable Integer Delay/1 -> Switch/1
  Ni--Lead/1 -> Variable Integer Delay/2
  Gain1/1 -> Subsystem1/1(In), Out/1
  Variable Integer Delay1/1 -> Sum18/2
  Discrete FIR/1 -> Gain1/1
  Saturation3/1 -> Discrete Filter1/1
  Seperated1/2(N) -> Sum4/2
  Saturation2/1 -> Mux/1, Sum4/1  "Ni"
  Sum4/1 -> Saturation3/1  "F"
  Seperated1/1(Ni) -> Saturation2/1
  f1/1 -> Seperated1/1(fi)
  Subsystem1/1(Out) -> Variable Integer Delay1/1
  Discrete Filter1/1 -> Subsystem1/2(F)
  Mux/1 -> Ni--Lead/1

== system Grid_PBFORCAPF_ab_Detail_2013b_616/Controller3/ICLARKE1 ==
  AB : Inport
  -0.5alfa+sqrt(3)/2*beta : Fcn  Expr=-u(1)/2+u(2)*sqrt(3)/2
  "-0.5alfa-sqrt(3)/2*beta " : Fcn  Expr=-u(1)/2-u(2)*sqrt(3)/2
  Mux3 : Mux  Inputs=3
  a=alfa : Fcn  Expr=u(1)
  ABC : Outport  VectorParamsAs1DForOutWhenUnconnected=off
  wires:
  -0.5alfa+sqrt(3)/2*beta/1 -> Mux3/2  "b"
  "-0.5alfa-sqrt(3)/2*beta "/1 -> Mux3/3  "c"
  Mux3/1 -> ABC/1
  AB/1 -> "-0.5alfa-sqrt(3)/2*beta "/1, -0.5alfa+sqrt(3)/2*beta/1, a=alfa/1
  a=alfa/1 -> Mux3/1  "a"

== system Grid_PBFORCAPF_ab_Detail_2013b_616/Controller3/IPARK ==
  dq : Inport
  Sin_Cos : Inport  Port=2
  Mux1 : Mux  Inputs=2
  Mux2 : Mux  Inputs=2
  cos*d-sin*q : Fcn  Expr=u(1)*u(4)-u(2)*u(3)
  sin*d+cos*q : Fcn  Expr=u(1)*u(3)+u(2)*u(4)
  AB : Outport  VectorParamsAs1DForOutWhenUnconnected=off
  wires:
  Mux2/1 -> cos*d-sin*q/1, sin*d+cos*q/1
  Sin_Cos/1 -> Mux2/2
  dq/1 -> Mux2/1
  cos*d-sin*q/1 -> Mux1/1
  sin*d+cos*q/1 -> Mux1/2  "beta"
  Mux1/1 -> AB/1

== system Grid_PBFORCAPF_ab_Detail_2013b_616/Controller3/SV Modulator Pattern #1 ==
  note: m_max
  note: 6/pi(2/sqrt(3)-1)=0.295
  Valphabeta : Inport
  Cartesian to Polar : simulink_extras/Transformations/Cartesian to Polar
  "Compute time duration of switching states (Ta,Tb,To) " : Subsystem
  Constant : Constant  Value=pi/3
  Constant2 : Constant  Value=2*pi
  Demux : Demux  Outputs=2
  "Determine the sector of U* based on alpha (rad). Also, determine if the sector number is odd" : Subsystem
  Generate pulse pattern : Subsystem
      mask init: same as Grid_PBFORCAPF_ab_Detail_2013b_616/Controller1/SV Modulator Pattern #1/Generate pulse pattern
  Hexagonal : Saturate  UpperLimit=0  LowerLimit=-10
  INFO : Subsystem
      mask Display: disp('?')
  Math Function : Math  Operator=reciprocal  SignedPower=on  SaturateOnIntegerOverflow=on
  Math Function2 : Math  Operator=mod  SignedPower=on  SaturateOnIntegerOverflow=on
  Mux : Mux  Inputs=2
  Polar to Cartesian : simulink_extras/Transformations/Polar to Cartesian
      settings: SourceProductBaseCode=SL
  Saturation : Saturate  UpperLimit=6  LowerLimit=1
  Subsystem : Subsystem
  Sum1 : Sum  Inputs=+-  SaturateOnIntegerOverflow=on
  Sum2 : Sum  SaturateOnIntegerOverflow=on
  Sum3 : Sum  SaturateOnIntegerOverflow=on
  Trigonometric Function : Trigonometry
  Dabc : Outport  VectorParamsAs1DForOutWhenUnconnected=off
  tag scope: Vsatab_DG3=global, Vunsatab_DG3=global
  wires:
  Math Function2/1 -> Polar to Cartesian/2, "Compute time duration of switching states (Ta,Tb,To) "/1(alpha), "Determine the sector of U* based on alpha (rad). Also, determine if the sector number is odd"/1(alpha)
  Generate pulse pattern/1(abc) -> Dabc/1
  "Compute time duration of switching states (Ta,Tb,To) "/1(Ta_Tb_To) -> Subsystem/1(TaTbTo)
  "Determine the sector of U* based on alpha (rad). Also, determine if the sector number is odd"/2(Odd_S) -> "Compute time duration of switching states (Ta,Tb,To) "/4(Odd_S)
  "Determine the sector of U* based on alpha (rad). Also, determine if the sector number is odd"/1(Sn) -> Saturation/1, "Compute time duration of switching states (Ta,Tb,To) "/3(Sn)
  Subsystem/1(D1D2D0) -> Generate pulse pattern/2(D120)
  Saturation/1 -> Generate pulse pattern/1(Sn)
  Demux/1 -> Cartesian to Polar/1
  Demux/2 -> Cartesian to Polar/2
  Cartesian to Polar/2 -> Math Function2/1
  Cartesian to Polar/1 -> Sum2/2, Sum1/2
  Constant2/1 -> Math Function2/2
  Sum2/1 -> Polar to Cartesian/1, "Compute time duration of switching states (Ta,Tb,To) "/2(m)
  Constant/1 -> Sum3/2
  [alpha3] -> Sum3/1
  Trigonometric Function/1 -> Math Function/1
  Sum1/1 -> Hexagonal/1
  Hexagonal/1 -> Sum2/1
  Polar to Cartesian/2 -> Mux/2
  Polar to Cartesian/1 -> Mux/1
  Mux/1 -> [Vsatab_DG3]
  Sum3/1 -> Trigonometric Function/1
  Math Function/1 -> Sum1/1
  Valphabeta/1 -> [Vunsatab_DG3], Demux/1

== system Grid_PBFORCAPF_ab_Detail_2013b_616/Measure/CLARKE ==
  ABC : Inport
  Fcn : Fcn  Expr=2/3*(u(1)-u(2)/2-u(3)/2)
  Fcn1 : Fcn  Expr=(u(2)-u(3))/sqrt(3)
  Mux : Mux  Inputs=2
  AB : Outport  VectorParamsAs1DForOutWhenUnconnected=off
  wires:
  ABC/1 -> Fcn1/1, Fcn/1
  Fcn/1 -> Mux/1  "alfa"
  Fcn1/1 -> Mux/2  "beta"
  Mux/1 -> AB/1

== system Grid_PBFORCAPF_ab_Detail_2013b_616/Measure/ICLARKE ==
  AB : Inport
  -0.5alfa+sqrt(3)/2*beta : Fcn  Expr=-u(1)/2+u(2)*sqrt(3)/2
  "-0.5alfa-sqrt(3)/2*beta " : Fcn  Expr=-u(1)/2-u(2)*sqrt(3)/2
  Mux3 : Mux  Inputs=3
  a=alfa : Fcn  Expr=u(1)
  ABC : Outport  VectorParamsAs1DForOutWhenUnconnected=off
  wires:
  a=alfa/1 -> Mux3/1  "a"
  AB/1 -> a=alfa/1, -0.5alfa+sqrt(3)/2*beta/1, "-0.5alfa-sqrt(3)/2*beta "/1
  Mux3/1 -> ABC/1
  "-0.5alfa-sqrt(3)/2*beta "/1 -> Mux3/3  "c"
  -0.5alfa+sqrt(3)/2*beta/1 -> Mux3/2  "b"

== system Grid_PBFORCAPF_ab_Detail_2013b_616/Measure/MSOGIs_A ==
  in : Inport
  Fcn : Fcn  Expr=u(1)
  Logical Operator1 : Logic  Operator=NOT  IconShape=distinctive  AllPortsSameDT=off  OutDataTypeStr=boolean
  RCA : Subsystem  mask{h=h, KIh=KIh, Ts=Ts}
      mask prompts: h "Selected harmonic orders"; KIh "Integral gain of SOGI"; Ts "Sampling Period"
      mask Display: disp('SOGIh(z)')
  Subtract : Sum  Inputs=+-
  Sum : Sum  Inputs=-+|
  Sum of Elements : Sum  Inputs=+
  Ihref : Outport  VectorParamsAs1DForOutWhenUnconnected=off
  wires:
  in/1 -> Sum/2
  Sum/1 -> RCA/1(v)
  [fpll] -> RCA/2(f0)
  [En_Meas] -> Logical Operator1/1
  RCA/1(vh) -> Fcn/1, Sum of Elements/1
  Sum of Elements/1 -> Subtract/1, Sum/1
  Logical Operator1/1 -> RCA/3(rest)
  Subtract/1 -> Ihref/1
  Fcn/1 -> Subtract/2

== system Grid_PBFORCAPF_ab_Detail_2013b_616/Measure/MSOGIs_B ==
  in : Inport
  Fcn : Fcn  Expr=u(1)
  Logical Operator1 : Logic  Operator=NOT  IconShape=distinctive  AllPortsSameDT=off  OutDataTypeStr=boolean
  RCA : Subsystem  mask{h=h, KIh=KIh, Ts=Ts}
      mask prompts: h "Selected harmonic orders"; KIh "Integral gain of SOGI"; Ts "Sampling Period"
      mask Display: disp('SOGIh(z)')
  Subtract : Sum  Inputs=+-
  Sum : Sum  Inputs=-+|
  Sum of Elements : Sum  Inputs=+
  Ihref : Outport  VectorParamsAs1DForOutWhenUnconnected=off
  wires:
  Fcn/1 -> Subtract/2
  Subtract/1 -> Ihref/1
  Logical Operator1/1 -> RCA/3(rest)
  Sum of Elements/1 -> Subtract/1, Sum/1
  RCA/1(vh) -> Fcn/1, Sum of Elements/1
  [En_Meas] -> Logical Operator1/1
  [fpll] -> RCA/2(f0)
  Sum/1 -> RCA/1(v)
  in/1 -> Sum/2

== system Grid_PBFORCAPF_ab_Detail_2013b_616/PLL/CLARKE ==
  ABC : Inport
  Fcn : Fcn  Expr=2/3*(u(1)-u(2)/2-u(3)/2)
  Fcn1 : Fcn  Expr=(u(2)-u(3))/sqrt(3)
  Mux : Mux  Inputs=2
  AB : Outport  VectorParamsAs1DForOutWhenUnconnected=off
  wires:
  Mux/1 -> AB/1
  Fcn1/1 -> Mux/2  "beta"
  Fcn/1 -> Mux/1  "alfa"
  ABC/1 -> Fcn/1, Fcn1/1

== system Grid_PBFORCAPF_ab_Detail_2013b_616/PLL/CLARKE1 ==
  ABC : Inport
  Fcn : Fcn  Expr=2/3*(u(1)-u(2)/2-u(3)/2)
  Fcn1 : Fcn  Expr=(u(2)-u(3))/sqrt(3)
  Mux : Mux  Inputs=2
  AB : Outport  VectorParamsAs1DForOutWhenUnconnected=off
  wires:
  ABC/1 -> Fcn1/1, Fcn/1
  Fcn/1 -> Mux/1  "alfa"
  Fcn1/1 -> Mux/2  "beta"
  Mux/1 -> AB/1

== system Grid_PBFORCAPF_ab_Detail_2013b_616/PLL/CLARKE2 ==
  ABC : Inport
  Fcn : Fcn  Expr=2/3*(u(1)-u(2)/2-u(3)/2)
  Fcn1 : Fcn  Expr=(u(2)-u(3))/sqrt(3)
  Mux : Mux  Inputs=2
  AB : Outport  VectorParamsAs1DForOutWhenUnconnected=off
  wires:
  Mux/1 -> AB/1
  Fcn1/1 -> Mux/2  "beta"
  Fcn/1 -> Mux/1  "alfa"
  ABC/1 -> Fcn/1, Fcn1/1

== system Grid_PBFORCAPF_ab_Detail_2013b_616/PLL/PARK ==
  AB : Inport
  Sin_Cos : Inport  Port=2
  -sin*alfa+cos*beta : Fcn  Expr=-u(1)*u(3)+u(2)*u(4)
  Mux1 : Mux  Inputs=2
  Mux2 : Mux  Inputs=2
  cos*alfa+sin*beta : Fcn  Expr=u(1)*u(4)+u(2)*u(3)
  dq : Outport  VectorParamsAs1DForOutWhenUnconnected=off
  wires:
  Mux1/1 -> dq/1
  cos*alfa+sin*beta/1 -> Mux1/1
  AB/1 -> Mux2/1
  -sin*alfa+cos*beta/1 -> Mux1/2
  Mux2/1 -> -sin*alfa+cos*beta/1, cos*alfa+sin*beta/1
  Sin_Cos/1 -> Mux2/2

== system Grid_PBFORCAPF_ab_Detail_2013b_616/PLL/PARK1 ==
  AB : Inport
  Sin_Cos : Inport  Port=2
  -sin*alfa+cos*beta : Fcn  Expr=-u(1)*u(3)+u(2)*u(4)
  Mux1 : Mux  Inputs=2
  Mux2 : Mux  Inputs=2
  cos*alfa+sin*beta : Fcn  Expr=u(1)*u(4)+u(2)*u(3)
  dq : Outport  VectorParamsAs1DForOutWhenUnconnected=off
  wires:
  Sin_Cos/1 -> Mux2/2
  Mux2/1 -> cos*alfa+sin*beta/1, -sin*alfa+cos*beta/1
  -sin*alfa+cos*beta/1 -> Mux1/2
  AB/1 -> Mux2/1
  cos*alfa+sin*beta/1 -> Mux1/1
  Mux1/1 -> dq/1

== system Grid_PBFORCAPF_ab_Detail_2013b_616/PLL/PARK2 ==
  AB : Inport
  Sin_Cos : Inport  Port=2
  -sin*alfa+cos*beta : Fcn  Expr=-u(1)*u(3)+u(2)*u(4)
  Mux1 : Mux  Inputs=2
  Mux2 : Mux  Inputs=2
  cos*alfa+sin*beta : Fcn  Expr=u(1)*u(4)+u(2)*u(3)
  dq : Outport  VectorParamsAs1DForOutWhenUnconnected=off
  wires:
  Mux1/1 -> dq/1
  cos*alfa+sin*beta/1 -> Mux1/1
  AB/1 -> Mux2/1
  -sin*alfa+cos*beta/1 -> Mux1/2
  Mux2/1 -> -sin*alfa+cos*beta/1, cos*alfa+sin*beta/1
  Sin_Cos/1 -> Mux2/2

== system Grid_PBFORCAPF_ab_Detail_2013b_616/PLL/Sin_Generater ==
  wi : Inport
  Add : Sum
  Constant : Constant  Value=2*pi  SampleTime=Tscon
  Gain2 : Gain  Gain=Ts_Control
  Math Function : Math  Operator=rem  SignedPower=on  SaturateOnIntegerOverflow=on
  Mux1 : Mux  Inputs=2
  Trigonometric Function2 : Trigonometry  Operator=cos
  Trigonometric Function3 : Trigonometry
  Unit Delay : UnitDelay  SampleTime=-1  HasFrameUpgradeWarning=on
  Sin_Cos : Outport  VectorParamsAs1DForOutWhenUnconnected=off
  wires:
  Mux1/1 -> Sin_Cos/1
  Trigonometric Function3/1 -> Mux1/1
  Trigonometric Function2/1 -> Mux1/2
  wi/1 -> Gain2/1
  Unit Delay/1 -> Add/2
  Add/1 -> Math Function/1
  Math Function/1 -> Unit Delay/1, Trigonometric Function2/1, Trigonometric Function3/1  "Theta"
  Constant/1 -> Math Function/2
  Gain2/1 -> Add/1

== system Grid_PBFORCAPF_ab_Detail_2013b_616/PLL/Sin_Generater1 ==
  wi : Inport
  Add : Sum
  Constant : Constant  Value=2*pi  SampleTime=Tscon
  Gain2 : Gain  Gain=Ts_Control
  Math Function : Math  Operator=rem  SignedPower=on  SaturateOnIntegerOverflow=on
  Mux1 : Mux  Inputs=2
  Trigonometric Function2 : Trigonometry  Operator=cos
  Trigonometric Function3 : Trigonometry
  Unit Delay : UnitDelay  SampleTime=-1  HasFrameUpgradeWarning=on
  Sin_Cos : Outport  VectorParamsAs1DForOutWhenUnconnected=off
  wires:
  Gain2/1 -> Add/1
  Constant/1 -> Math Function/2
  Math Function/1 -> Trigonometric Function3/1, Trigonometric Function2/1, Unit Delay/1  "Theta"
  Add/1 -> Math Function/1
  Unit Delay/1 -> Add/2
  wi/1 -> Gain2/1
  Trigonometric Function2/1 -> Mux1/2
  Trigonometric Function3/1 -> Mux1/1
  Mux1/1 -> Sin_Cos/1

== system Grid_PBFORCAPF_ab_Detail_2013b_616/PLL/Sin_Generater2 ==
  wi : Inport
  Add : Sum
  Constant : Constant  Value=2*pi  SampleTime=Tscon
  Gain2 : Gain  Gain=Ts_Control
  Math Function : Math  Operator=rem  SignedPower=on  SaturateOnIntegerOverflow=on
  Mux1 : Mux  Inputs=2
  Trigonometric Function2 : Trigonometry  Operator=cos
  Trigonometric Function3 : Trigonometry
  Unit Delay : UnitDelay  SampleTime=-1  HasFrameUpgradeWarning=on
  Sin_Cos : Outport  VectorParamsAs1DForOutWhenUnconnected=off
  wires:
  Mux1/1 -> Sin_Cos/1
  Trigonometric Function3/1 -> Mux1/1
  Trigonometric Function2/1 -> Mux1/2
  wi/1 -> Gain2/1
  Unit Delay/1 -> Add/2
  Add/1 -> Math Function/1
  Math Function/1 -> Unit Delay/1, Trigonometric Function2/1, Trigonometric Function3/1  "Theta"
  Constant/1 -> Math Function/2
  Gain2/1 -> Add/1

== system Grid_PBFORCAPF_ab_Detail_2013b_616/Controller1/DSOGI/QSOGI ==
  v : Inport
  2 : Gain  Gain=2
  2*pi*h*Ts : Gain  Gain=6.28*h*Ts
  Constant : Constant  SampleTime=Tscon
  Constant1 : Constant  Value=50  SampleTime=Tscon
  Discrete-Time Integrator : DiscreteIntegrator  IntegratorMethod=Accumulation: Backward Euler  SampleTime=-1  ICPrevOutput=DiscIntNeverNeededParam  ICPrevScaledInput=DiscIntNeverNeededParam
  Discrete-Time Integrator1 : DiscreteIntegrator  IntegratorMethod=Accumulation: Forward Euler  SampleTime=-1  ICPrevOutput=DiscIntNeverNeededParam  ICPrevScaledInput=DiscIntNeverNeededParam
  KIh : Gain  Gain=KIh*Ts
  Product1 : Product
  Sum1 : Sum  Inputs=|+-
  Sum2 : Sum  Inputs=|+-
  Sum3 : Sum  Inputs=-+|
  Sum4 : Sum  Inputs=|++
  Sum5 : Sum  Inputs=|++
  cos(314*h*Ts)-1 : Gain  Gain=cos(314*h*Ts)-1
  cos(314*h*Ts+phch)-cos(phch) : Gain  Gain=cos(314*h*Ts+phch)-cos(phch)
  cos(phch) : Gain  Gain=cos(phch)
  cos(wh*Ts) : Trigonometry  Operator=cos
  wc : Gain  Gain=wc
  vh : Outport  VectorParamsAs1DForOutWhenUnconnected=off
  wires:
  Product1/1 -> Sum2/2
  Sum2/1 -> Discrete-Time Integrator1/1
  v/1 -> Sum3/2
  KIh/1 -> Sum2/1
  Constant1/1 -> 2*pi*h*Ts/1
  Discrete-Time Integrator1/1 -> Discrete-Time Integrator/1, cos(phch)/1, Sum5/2
  Discrete-Time Integrator/1 -> cos(314*h*Ts)-1/1, cos(314*h*Ts+phch)-cos(phch)/1, Product1/2
  2*pi*h*Ts/1 -> cos(wh*Ts)/1
  cos(wh*Ts)/1 -> Sum1/2
  Constant/1 -> Sum1/1
  Sum1/1 -> 2/1
  2/1 -> Product1/1
  cos(phch)/1 -> Sum4/1
  cos(314*h*Ts+phch)-cos(phch)/1 -> Sum4/2
  Sum4/1 -> vh/1
  wc/1 -> Sum3/1
  Sum3/1 -> KIh/1
  Sum5/1 -> wc/1
  cos(314*h*Ts)-1/1 -> Sum5/1

== system Grid_PBFORCAPF_ab_Detail_2013b_616/Controller1/FORCAB/Seperated1 ==
  fi : Inport
  Compare To Constant : simulink/Logic and Bit Operations/Compare To Constant  relop=>=  const=50  OutDataTypeStr=boolean
  Compare To Constant1 : simulink/Logic and Bit Operations/Compare To Constant  relop=<  const=-10  OutDataTypeStr=boolean
  Constant : Constant  Value=1/Ts_Control  SampleTime=Tscon
  Data Type Conversion : DataTypeConversion  OutDataTypeStr=double
  Data Type Conversion1 : DataTypeConversion  OutDataTypeStr=double
  Discrete-Time Integrator : DiscreteIntegrator  gainval=1/Ts_Control  ExternalReset=level  InitialCondition=200  SampleTime=-1  LimitOutput=on  UpperSaturationLimit=300  LowerSaturationLimit=100  ICPrevOutput=DiscIntNeverNeededParam  ICPrevScaledInput=DiscIntNeverNeededParam
  N=1/f0/Ts : Fcn  Expr=1/u(1)/Ts
  Product2 : Product
  Sum3 : Sum  Inputs=+-
  Sum4 : Sum  Inputs=+-
  Ni : Outport  VectorParamsAs1DForOutWhenUnconnected=off
  N : Outport  Port=2  VectorParamsAs1DForOutWhenUnconnected=off
  wires:
  Product2/1 -> Sum3/2
  Constant/1 -> Sum3/1
  N=1/f0/Ts/1 -> N/1
  Sum4/1 -> Discrete-Time Integrator/1
  Data Type Conversion1/1 -> Sum4/2
  Compare To Constant1/1 -> Data Type Conversion1/1
  fi/1 -> N=1/f0/Ts/1, Product2/1
  Sum3/1 -> Compare To Constant/1, Compare To Constant1/1
  Compare To Constant/1 -> Data Type Conversion/1
  [RSTT1] -> Discrete-Time Integrator/2
  Discrete-Time Integrator/1 -> Ni/1, Product2/2  "Ni2"
  Data Type Conversion/1 -> Sum4/1

== system Grid_PBFORCAPF_ab_Detail_2013b_616/Controller1/FORCAB/Subsystem1 ==
  In : Inport
  F : Inport  Port=2
  1-F : Fcn  Expr=1-u(1)
  Product : Product
  Product1 : Product
  Sum3 : Sum
  Unit Delay1 : UnitDelay  SampleTime=-1  HasFrameUpgradeWarning=on
  Out : Outport  VectorParamsAs1DForOutWhenUnconnected=off
  wires:
  F/1 -> 1-F/1, Product/2
  Product/1 -> Sum3/1
  In/1 -> Product1/1, Unit Delay1/1
  1-F/1 -> Product1/2
  Sum3/1 -> Out/1
  Unit Delay1/1 -> Product/1
  Product1/1 -> Sum3/2

== system Grid_PBFORCAPF_ab_Detail_2013b_616/Controller1/SV Modulator Pattern #1/Compute time duration of switching states (Ta,Tb,To)  ==
  note: TaTbTo
  note: To=(1/Fc-Ta-Tb)
  note: Tb=m*sin(alpha) * (1/Fc)
  note: Ta=m*cos(alpha+30)* (1/Fc)
  alpha : Inport
  m : Inport  Port=2
  Sn : Inport  Port=3
  Odd_S : Inport  Port=4
  Constant : Constant  Value=pi/6
  Constant1 : Constant  Value=pi/3
  Constant2 : Constant
  Constant8 : Constant
  Mux : Mux  Inputs=2
  Mux1 : Mux  Inputs=2
  Product : Product  SaturateOnIntegerOverflow=on  OutDataTypeStr=Inherit: Same as first input
  Product1 : Product  SaturateOnIntegerOverflow=on  OutDataTypeStr=Inherit: Same as first input
  Selector1 : Selector  InputPortWidth=3  IndexOptions=Index vector (dialog)  Indices=[2 1 3]  OutputSizes=1
  Sum : Sum  SaturateOnIntegerOverflow=on
  Sum1 : Sum  Inputs=+-  SaturateOnIntegerOverflow=on
  Sum2 : Sum  Inputs=1  SaturateOnIntegerOverflow=on
  Sum3 : Sum  Inputs=-+  SaturateOnIntegerOverflow=on
  Sum4 : Sum  Inputs=+-  SaturateOnIntegerOverflow=on
  Switch1 : Switch  Threshold=0.5  SaturateOnIntegerOverflow=on
  Trigonometric Function : Trigonometry
  Trigonometric Function1 : Trigonometry  Operator=cos
  Ta_Tb_To : Outport  VectorParamsAs1DForOutWhenUnconnected=off
  tag scope: alpha=global
  wires:
  Odd_S/1 -> Switch1/2
  Switch1/1 -> Ta_Tb_To/1
  Selector1/1 -> Switch1/3
  Mux1/1 -> Selector1/1, Switch1/1
  Constant/1 -> Sum/2
  Sum4/1 -> [alpha], Trigonometric Function/1, Sum/1  "alpha"
  Sum3/1 -> Mux1/2  "To"
  Product/1 -> Sum2/1, Mux1/1  "TaTb"
  alpha/1 -> Sum4/1
  Product1/1 -> Sum4/2
  Constant2/1 -> Sum1/2
  Sn/1 -> Sum1/1
  Constant1/1 -> Product1/2
  Sum1/1 -> Product1/1
  Constant8/1 -> Sum3/2
  Sum2/1 -> Sum3/1
  Sum/1 -> Trigonometric Function1/1
  m/1 -> Product/1
  Mux/1 -> Product/2
  Trigonometric Function/1 -> Mux/2
  Trigonometric Function1/1 -> Mux/1
